simulink model "dmitry_model"  (R2022b)
settings: Solver=FixedStepDiscrete  StartTime=0.0  StopTime=10.0  FixedStep=1/ SCHED_LOOP_RATE  RelTol=1e-3
values from neighbouring files (symbols this model uses):
  g = 9.81    [startVars.m]
  KDphi = KDphi*1.0    (= 0.00082498)    [altitude_attitude_control_sim.m]
  KDpsi = KDpsi*1.0*0.8    (= 0.0004576)    [altitude_attitude_control_sim.m]
  KDtheta = KDtheta*1.4    (= 0.001977976)    [altitude_attitude_control_sim.m]
  KDz = KDz*1.0    (= 0.3498)    [altitude_attitude_control_sim.m]
  Ts = 1/SCHED_LOOP_RATE    [PitchComplementaryFilter_disc.m]    (also in RollComplementaryFilter_disc.m; YawComplementaryFilter_disc.m; altitude_attitude_control_sim.m; startVars.m)
  w_c_pitch = 0.3    [PitchComplementaryFilter_disc.m]
  w_c_roll = 0.3    [RollComplementaryFilter_disc.m]
  w_c_yaw = 55    [YawComplementaryFilter_disc.m]
  zDphi = zDphi*1.0    (= 1.31578947368)    [altitude_attitude_control_sim.m]
  zDpsi = zDpsi*1.0*1.0    (= 2.27272727273)    [altitude_attitude_control_sim.m]
  zDtheta = zDtheta*1.0    (= 1.31578947368)    [altitude_attitude_control_sim.m]
  zDz = zDz*1.0    (= 3.0303030303)    [altitude_attitude_control_sim.m]
undefined symbols (not defined in the file or in its folder): Controller, den_pitch_disc, den_roll_disc, den_yaw_disc, num_pitch_disc, num_roll_disc, num_yaw_disc, Vehicle
libraries: cstblocks x9
settings Model: ParamWorkspaceSource=ReferencedWorkspace  Creator=joseph  LastModifiedBy=Joseph
settings OptimizationCC: EnhancedBackFolding=on  PassReuseOutputArgsAs=Individual arguments  ZeroExternalMemoryAtStartup=off  ZeroInternalMemoryAtStartup=off  OptimizeBlockOrder=speed  DifferentSizesBufferReuse=on  OptimizationCustomize=off  EfficientTunableParamExpr=on
settings DebuggingCC: ParameterTunabilityLossMsg=error
settings HardwareCC: ProdBitPerPointer=32  ProdBitPerSizeT=32  ProdBitPerPtrDiffT=32  ProdLargestAtomicInteger=Long  ProdLargestAtomicFloat=Double  ProdWordSize=32  ProdHWDeviceType=ARM Compatible->ARM Cortex-M
settings SFSimCC: MATLABDynamicMemAlloc=off
settings RTWCC: Description=Embedded Coder  SystemTargetFile=ert.tlc  GenCodeOnly=on  PackageGeneratedCodeAndArtifacts=on  TemplateMakefile=ert_default_tmf  Toolchain=MinGW64 | gmake (64-bit Windows)  TargetLang=C++
settings CodeAppCC: ForceParamTrailComments=on  IgnoreCustomStorageClasses=off  OperatorAnnotations=on  SimulinkDataObjDesc=on  SFDataObjDesc=on  InsertBlockDesc=on
settings ERTTargetCC: TargetLangStandard=C++11 (ISO)  GenerateSampleERTMain=on  CodeInterfacePackaging=C++ class  RootIOFormat=Structure reference  ERTCustomFileTemplate=example_file_process.tlc

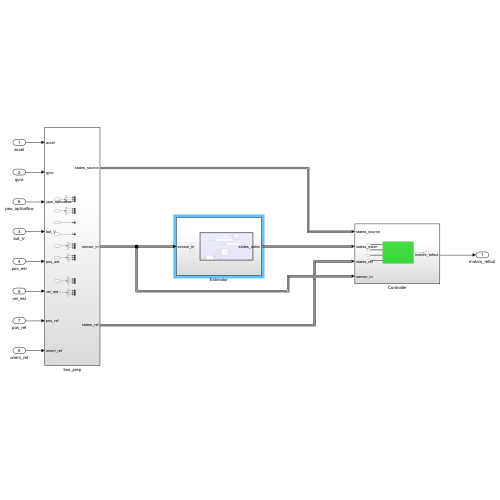
[thumbnail: Simulink's stored preview of the top-level diagram]
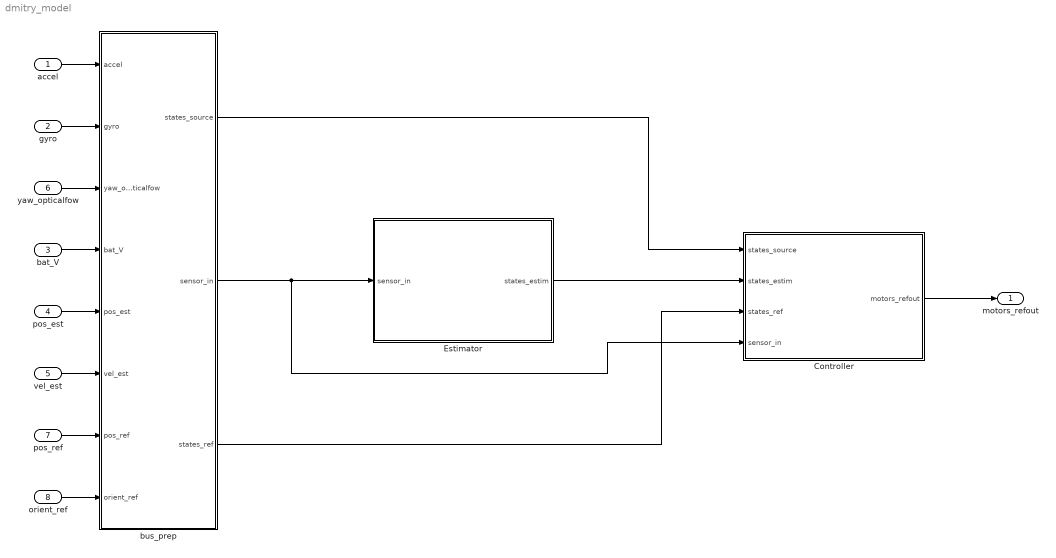
== system dmitry_model ==
  accel : Inport  OutDataTypeStr=single
  gyro : Inport  Port=2  OutDataTypeStr=single
  bat_V : Inport  Port=3  OutDataTypeStr=single
  pos_est : Inport  Port=4  OutDataTypeStr=single
  vel_est : Inport  Port=5  OutDataTypeStr=single
  yaw_opticalfow : Inport  Port=6  OutDataTypeStr=single
  pos_ref : Inport  Port=7  OutDataTypeStr=single
  orient_ref : Inport  Port=8  OutDataTypeStr=single
  Controller : Subsystem
  Estimator : Subsystem
  bus_prep : Subsystem
  motors_refout : Outport
  wires:
  accel/1 -> bus_prep/1(accel)
  gyro/1 -> bus_prep/2(gyro)
  yaw_opticalfow/1 -> bus_prep/3(yaw_opticalfow)
  bat_V/1 -> bus_prep/4(bat_V)
  pos_est/1 -> bus_prep/5(pos_est)
  vel_est/1 -> bus_prep/6(vel_est)
  pos_ref/1 -> bus_prep/7(pos_ref)
  orient_ref/1 -> bus_prep/8(orient_ref)
  bus_prep/2(sensor_in) -> Controller/4(sensor_in), Estimator/1(sensor_in)
  bus_prep/1(states_source) -> Controller/1(states_source)
  Estimator/1(states_estim) -> Controller/2(states_estim)
  Controller/1(motors_refout) -> motors_refout/1
  bus_prep/3(states_ref) -> Controller/3(states_ref)

== system dmitry_model/Controller ==
  states_source : Inport
  states_estim : Inport  Port=2
  states_ref : Inport  Port=3
  sensor_in : Inport  Port=4
  Flight Controller : Subsystem
  motors_refout : Outport
  wires:
  Flight Controller/1(motors_refout) -> motors_refout/1
  states_ref/1 -> Flight Controller/3(states_ref)
  states_estim/1 -> Flight Controller/2(states_est)
  states_source/1 -> Flight Controller/1(states_source)
  sensor_in/1 -> Flight Controller/4(sensor_in)

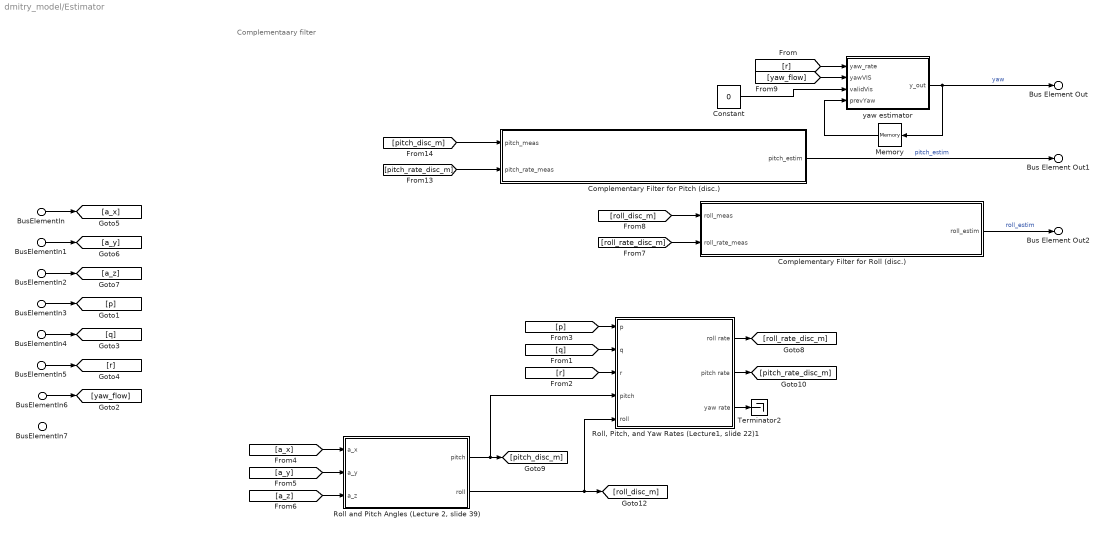
== system dmitry_model/Estimator ==
  note: Complementaary filter
  BusElementIn : Inport  PortName=sensor_in  Element=a_x
  BusElementIn1 : Inport  PortName=sensor_in  Element=a_y
  BusElementIn2 : Inport  PortName=sensor_in  Element=a_z
  BusElementIn3 : Inport  PortName=sensor_in  Element=p
  BusElementIn4 : Inport  PortName=sensor_in  Element=q
  BusElementIn5 : Inport  PortName=sensor_in  Element=r
  BusElementIn6 : Inport  PortName=sensor_in  Element=yaw_flow
  BusElementIn7 : Inport  PortName=sensor_in  Element=yaw_flow
  Complementary Filter for Pitch (disc.) : Subsystem
  Complementary Filter for Roll (disc.) : Subsystem
  Constant : Constant  Value=0
  Memory : Memory
  "Roll and Pitch Angles (Lecture 2, slide 39)" : Subsystem
  "Roll, Pitch, and Yaw Rates (Lecture1, slide 22)1" : Subsystem
  Terminator2 : Terminator
  yaw estimator : Subsystem
  Bus Element Out : Outport  PortName=states_estim  Element=yaw
  Bus Element Out1 : Outport  PortName=states_estim  Element=pitch
  Bus Element Out2 : Outport  PortName=states_estim  Element=roll
  wires:
  [a_y] -> "Roll and Pitch Angles (Lecture 2, slide 39)"/2(a_y)
  [p] -> "Roll, Pitch, and Yaw Rates (Lecture1, slide 22)1"/1(p)
  [a_x] -> "Roll and Pitch Angles (Lecture 2, slide 39)"/1(a_x)
  "Roll and Pitch Angles (Lecture 2, slide 39)"/2(roll) -> "Roll, Pitch, and Yaw Rates (Lecture1, slide 22)1"/5(roll), [roll_disc_m]
  [a_z] -> "Roll and Pitch Angles (Lecture 2, slide 39)"/3(a_z)
  "Roll and Pitch Angles (Lecture 2, slide 39)"/1(pitch) -> [pitch_disc_m], "Roll, Pitch, and Yaw Rates (Lecture1, slide 22)1"/4(pitch)
  Constant/1 -> yaw estimator/3(validVis)
  [roll_rate_disc_m] -> Complementary Filter for Roll (disc.)/2(roll_rate_meas)
  [roll_disc_m] -> Complementary Filter for Roll (disc.)/1(roll_meas)
  Complementary Filter for Roll (disc.)/1(roll_estim) -> Bus Element Out2/1  "roll_estim"
  [q] -> "Roll, Pitch, and Yaw Rates (Lecture1, slide 22)1"/2(q)
  "Roll, Pitch, and Yaw Rates (Lecture1, slide 22)1"/3(yaw rate) -> Terminator2/1
  "Roll, Pitch, and Yaw Rates (Lecture1, slide 22)1"/2(pitch rate) -> [pitch_rate_disc_m]
  Complementary Filter for Pitch (disc.)/1(pitch_estim) -> Bus Element Out1/1  "pitch_estim"
  [r] -> "Roll, Pitch, and Yaw Rates (Lecture1, slide 22)1"/3(r)
  [yaw_flow] -> yaw estimator/2(yawVIS)
  [pitch_disc_m] -> Complementary Filter for Pitch (disc.)/1(pitch_meas)
  Memory/1 -> yaw estimator/4(prevYaw)
  [pitch_rate_disc_m] -> Complementary Filter for Pitch (disc.)/2(pitch_rate_meas)
  yaw estimator/1(y_out) -> Bus Element Out/1, Memory/1  "yaw"
  "Roll, Pitch, and Yaw Rates (Lecture1, slide 22)1"/1(roll rate) -> [roll_rate_disc_m]
  [r] -> yaw estimator/1(yaw_rate)
  BusElementIn3/1 -> [p]
  BusElementIn4/1 -> [q]
  BusElementIn5/1 -> [r]
  BusElementIn/1 -> [a_x]
  BusElementIn1/1 -> [a_y]
  BusElementIn2/1 -> [a_z]
  BusElementIn6/1 -> [yaw_flow]

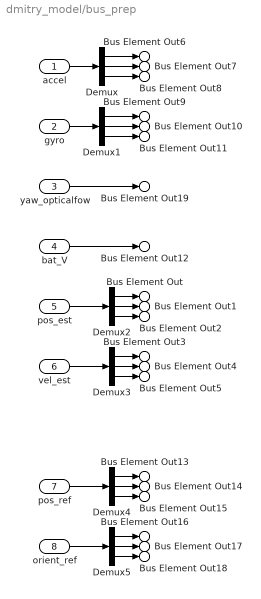
== system dmitry_model/bus_prep ==
  accel : Inport  OutDataTypeStr=single
  gyro : Inport  Port=2  OutDataTypeStr=single
  yaw_opticalfow : Inport  Port=3  OutDataTypeStr=single
  bat_V : Inport  Port=4  OutDataTypeStr=single
  pos_est : Inport  Port=5  OutDataTypeStr=single
  vel_est : Inport  Port=6  OutDataTypeStr=single
  pos_ref : Inport  Port=7  OutDataTypeStr=single
  orient_ref : Inport  Port=8  OutDataTypeStr=single
  Demux{,1..5} (6 alike) : Demux  Outputs=3
  Bus Element Out : Outport  PortName=states_source  Element=x
  Bus Element Out1 : Outport  PortName=states_source  Element=y
  Bus Element Out2 : Outport  PortName=states_source  Element=z
  Bus Element Out3 : Outport  PortName=states_source  Element=dx
  Bus Element Out4 : Outport  PortName=states_source  Element=dy
  Bus Element Out5 : Outport  PortName=states_source  Element=dz
  Bus Element Out6 : Outport  Port=2  PortName=sensor_in  Element=a_x
  Bus Element Out7 : Outport  Port=2  PortName=sensor_in  Element=a_y
  Bus Element Out8 : Outport  Port=2  PortName=sensor_in  Element=a_z
  Bus Element Out9 : Outport  Port=2  PortName=sensor_in  Element=p
  Bus Element Out10 : Outport  Port=2  PortName=sensor_in  Element=q
  Bus Element Out11 : Outport  Port=2  PortName=sensor_in  Element=r
  Bus Element Out12 : Outport  Port=2  PortName=sensor_in  Element=V_batt
  Bus Element Out19 : Outport  Port=2  PortName=sensor_in  Element=yaw_flow
  Bus Element Out13 : Outport  Port=3  PortName=states_ref  Element=x
  Bus Element Out14 : Outport  Port=3  PortName=states_ref  Element=y
  Bus Element Out15 : Outport  Port=3  PortName=states_ref  Element=z
  Bus Element Out16 : Outport  Port=3  PortName=states_ref  Element=yaw
  Bus Element Out17 : Outport  Port=3  PortName=states_ref  Element=pitch
  Bus Element Out18 : Outport  Port=3  PortName=states_ref  Element=roll
  wires:
  pos_ref/1 -> Demux4/1
  orient_ref/1 -> Demux5/1
  pos_est/1 -> Demux2/1
  Demux3/1 -> Bus Element Out3/1
  Demux3/3 -> Bus Element Out5/1
  Demux5/3 -> Bus Element Out18/1
  vel_est/1 -> Demux3/1
  accel/1 -> Demux/1
  gyro/1 -> Demux1/1
  Demux5/1 -> Bus Element Out16/1
  Demux4/1 -> Bus Element Out13/1
  Demux1/1 -> Bus Element Out9/1
  Demux3/2 -> Bus Element Out4/1
  Demux4/2 -> Bus Element Out14/1
  Demux2/2 -> Bus Element Out1/1
  Demux1/3 -> Bus Element Out11/1
  Demux5/2 -> Bus Element Out17/1
  Demux4/3 -> Bus Element Out15/1
  Demux2/1 -> Bus Element Out/1
  Demux/3 -> Bus Element Out8/1
  Demux/1 -> Bus Element Out6/1
  Demux2/3 -> Bus Element Out2/1
  Demux1/2 -> Bus Element Out10/1
  yaw_opticalfow/1 -> Bus Element Out19/1
  bat_V/1 -> Bus Element Out12/1
  Demux/2 -> Bus Element Out7/1

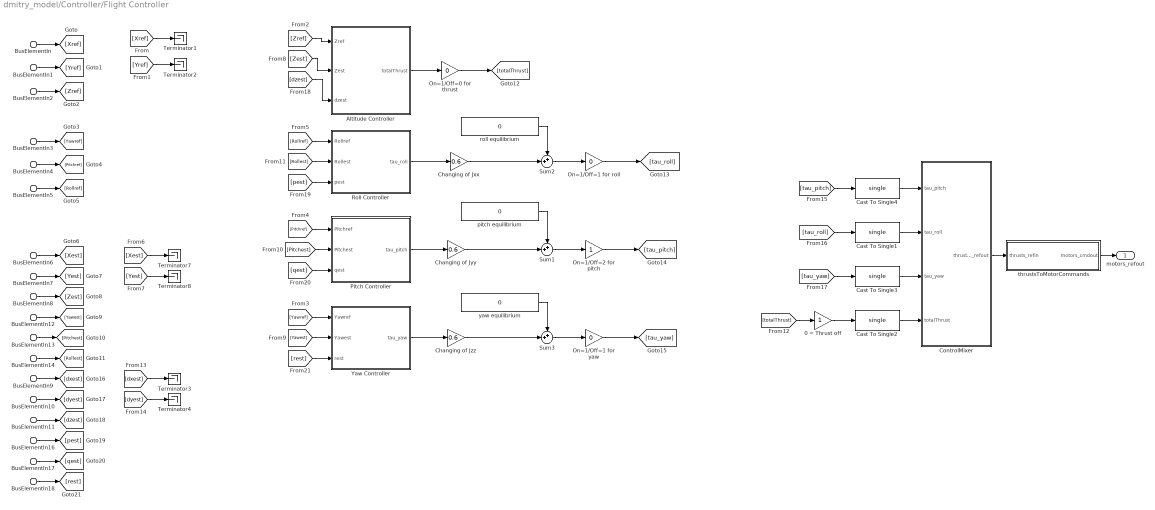
== system dmitry_model/Controller/Flight Controller ==
  BusElementIn6 : Inport  PortName=states_source  Element=x
  BusElementIn7 : Inport  PortName=states_source  Element=y
  BusElementIn8 : Inport  PortName=states_source  Element=z
  BusElementIn9 : Inport  PortName=states_source  Element=dx
  BusElementIn10 : Inport  PortName=states_source  Element=dy
  BusElementIn11 : Inport  PortName=states_source  Element=dz
  BusElementIn12 : Inport  Port=2  PortName=states_est  Element=yaw
  BusElementIn13 : Inport  Port=2  PortName=states_est  Element=pitch
  BusElementIn14 : Inport  Port=2  PortName=states_est  Element=roll
  BusElementIn : Inport  Port=3  PortName=states_ref  Element=x
  BusElementIn1 : Inport  Port=3  PortName=states_ref  Element=y
  BusElementIn2 : Inport  Port=3  PortName=states_ref  Element=z
  BusElementIn3 : Inport  Port=3  PortName=states_ref  Element=yaw
  BusElementIn4 : Inport  Port=3  PortName=states_ref  Element=pitch
  BusElementIn5 : Inport  Port=3  PortName=states_ref  Element=roll
  BusElementIn16 : Inport  Port=4  PortName=sensor_in  Element=p
  BusElementIn17 : Inport  Port=4  PortName=sensor_in  Element=q
  BusElementIn18 : Inport  Port=4  PortName=sensor_in  Element=r
  0 = Thrust off : Gain
  Altitude Controller : Subsystem
  Cast To Single{1..4} (4 alike) : DataTypeConversion  OutDataTypeStr=single  SaturateOnIntegerOverflow=off  RndMeth=Floor
  Changing of Jxx : Gain  Gain=0.6
  Changing of Jyy : Gain  Gain=0.6
  Changing of Jzz : Gain  Gain=0.6
  ControlMixer : Subsystem
  On=1/Off=0 for thrust : Gain  Gain=0
  On=1/Off=1 for roll : Gain  Gain=0
  On=1/Off=1 for yaw : Gain  Gain=0
  On=1/Off=2 for pitch : Gain
  Pitch Controller : Subsystem
  Roll Controller : Subsystem
  Sum1 : Sum  Inputs=++|
  Sum2 : Sum  Inputs=++|
  Sum3 : Sum  Inputs=++|
  Terminator{1..4,7..8} (6 alike) : Terminator
  Yaw Controller : Subsystem
  pitch equilibrium : Constant  Value=0  SampleTime=Ts
  roll equilibrium : Constant  Value=0  SampleTime=Ts
  thrustsToMotorCommands : Subsystem
  yaw equilibrium : Constant  Value=0  SampleTime=Ts
  motors_refout : Outport  VectorParamsAs1DForOutWhenUnconnected=off
  wires:
  ControlMixer/1(thrusts_refout) -> thrustsToMotorCommands/1(thrusts_refin)
  thrustsToMotorCommands/1(motors_cmdout) -> motors_refout/1
  Cast To Single1/1 -> ControlMixer/2(tau_roll)
  [tau_roll] -> Cast To Single1/1
  Cast To Single2/1 -> ControlMixer/4(totalThrust)
  BusElementIn/1 -> [Xref]
  BusElementIn1/1 -> [Yref]
  BusElementIn2/1 -> [Zref]
  BusElementIn5/1 -> [Rollref]
  BusElementIn4/1 -> [Pitchref]
  BusElementIn3/1 -> [Yawref]
  [Xref] -> Terminator1/1
  [Yref] -> Terminator2/1
  [Zref] -> Altitude Controller/1(Zref)
  BusElementIn6/1 -> [Xest]
  BusElementIn7/1 -> [Yest]
  BusElementIn8/1 -> [Zest]
  BusElementIn12/1 -> [Yawest]
  BusElementIn13/1 -> [Pitchest]
  BusElementIn14/1 -> [Rollest]
  [Zest] -> Altitude Controller/2(Zest)
  [Yest] -> Terminator8/1
  [Xest] -> Terminator7/1
  Altitude Controller/1(totalThrust) -> On=1/Off=0 for thrust/1
  On=1/Off=0 for thrust/1 -> [totalThrust]
  [totalThrust] -> 0 = Thrust off/1
  Roll Controller/1(tau_roll) -> Changing of Jxx/1
  [tau_yaw] -> Cast To Single3/1
  Cast To Single3/1 -> ControlMixer/3(tau_yaw)
  [tau_pitch] -> Cast To Single4/1
  Cast To Single4/1 -> ControlMixer/1(tau_pitch)
  [Rollref] -> Roll Controller/1(Rollref)
  [Rollest] -> Roll Controller/2(Rollest)
  Pitch Controller/1(tau_pitch) -> Changing of Jyy/1
  [Pitchest] -> Pitch Controller/2(Pitchest)
  [Pitchref] -> Pitch Controller/1(Pitchref)
  Yaw Controller/1(tau_yaw) -> Changing of Jzz/1
  [Yawref] -> Yaw Controller/1(Yawref)
  [Yawest] -> Yaw Controller/2(Yawest)
  BusElementIn9/1 -> [dxest]
  BusElementIn10/1 -> [dyest]
  BusElementIn11/1 -> [dzest]
  BusElementIn16/1 -> [pest]
  BusElementIn17/1 -> [qest]
  BusElementIn18/1 -> [rest]
  [dxest] -> Terminator3/1
  [dyest] -> Terminator4/1
  [pest] -> Roll Controller/3(pest)
  [dzest] -> Altitude Controller/3(dzest)
  [qest] -> Pitch Controller/3(qest)
  [rest] -> Yaw Controller/3(rest)
  roll equilibrium/1 -> Sum2/1
  Changing of Jxx/1 -> Sum2/2
  pitch equilibrium/1 -> Sum1/1
  yaw equilibrium/1 -> Sum3/1
  Changing of Jyy/1 -> Sum1/2
  Changing of Jzz/1 -> Sum3/2
  Sum3/1 -> On=1/Off=1 for yaw/1
  Sum1/1 -> On=1/Off=2 for pitch/1
  Sum2/1 -> On=1/Off=1 for roll/1
  On=1/Off=1 for roll/1 -> [tau_roll]
  On=1/Off=2 for pitch/1 -> [tau_pitch]
  On=1/Off=1 for yaw/1 -> [tau_yaw]
  0 = Thrust off/1 -> Cast To Single2/1

== system dmitry_model/Estimator/Complementary Filter for Pitch (disc.) ==
  pitch_meas : Inport
  pitch_rate_meas : Inport  Port=2
  Discrete Transfer Fcn : DiscreteTransferFcn  Numerator=[num_pitch_disc]  Denominator=[den_pitch_disc]  SampleTime=Ts
  Gain : Gain  Gain=w_c_pitch
  Sum : Sum  Inputs=+|+
  pitch_estim : Outport
  wires:
  Sum/1 -> Discrete Transfer Fcn/1
  Gain/1 -> Sum/1
  pitch_rate_meas/1 -> Sum/2
  pitch_meas/1 -> Gain/1
  Discrete Transfer Fcn/1 -> pitch_estim/1  "pitch_estim"

== system dmitry_model/Estimator/Complementary Filter for Roll (disc.) ==
  roll_meas : Inport
  roll_rate_meas : Inport  Port=2
  Discrete Transfer Fcn : DiscreteTransferFcn  Numerator=[num_roll_disc]  Denominator=[den_roll_disc]  SampleTime=Ts
  Gain : Gain  Gain=w_c_roll
  Sum : Sum  Inputs=+|+
  roll_estim : Outport
  wires:
  Discrete Transfer Fcn/1 -> roll_estim/1  "roll_estim"
  roll_meas/1 -> Gain/1
  roll_rate_meas/1 -> Sum/2
  Gain/1 -> Sum/1
  Sum/1 -> Discrete Transfer Fcn/1

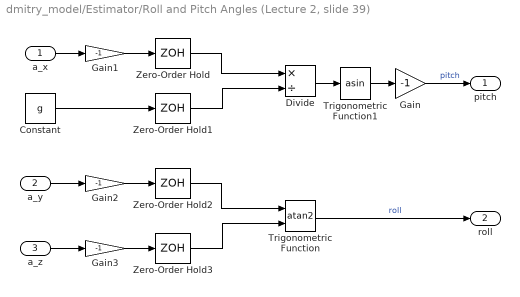
== system dmitry_model/Estimator/Roll and Pitch Angles (Lecture 2, slide 39) ==
  a_x : Inport
  a_y : Inport  Port=2
  a_z : Inport  Port=3
  Constant : Constant  Value=g
  Divide : Product  Inputs=*/
  Gain{,1..3} (4 alike) : Gain  Gain=-1
  Trigonometric Function : Trigonometry  Operator=atan2
  Trigonometric Function1 : Trigonometry  Operator=asin
  Zero-Order Hold{,1..3} (4 alike) : ZeroOrderHold  SampleTime=Ts
  pitch : Outport
  roll : Outport  Port=2
  wires:
  Gain/1 -> pitch/1  "pitch"
  Trigonometric Function/1 -> roll/1  "roll"
  a_y/1 -> Gain2/1
  a_z/1 -> Gain3/1
  a_x/1 -> Gain1/1
  Constant/1 -> Zero-Order Hold1/1
  Trigonometric Function1/1 -> Gain/1
  Divide/1 -> Trigonometric Function1/1
  Zero-Order Hold/1 -> Divide/1
  Zero-Order Hold1/1 -> Divide/2
  Zero-Order Hold2/1 -> Trigonometric Function/1
  Zero-Order Hold3/1 -> Trigonometric Function/2
  Gain1/1 -> Zero-Order Hold/1
  Gain2/1 -> Zero-Order Hold2/1
  Gain3/1 -> Zero-Order Hold3/1

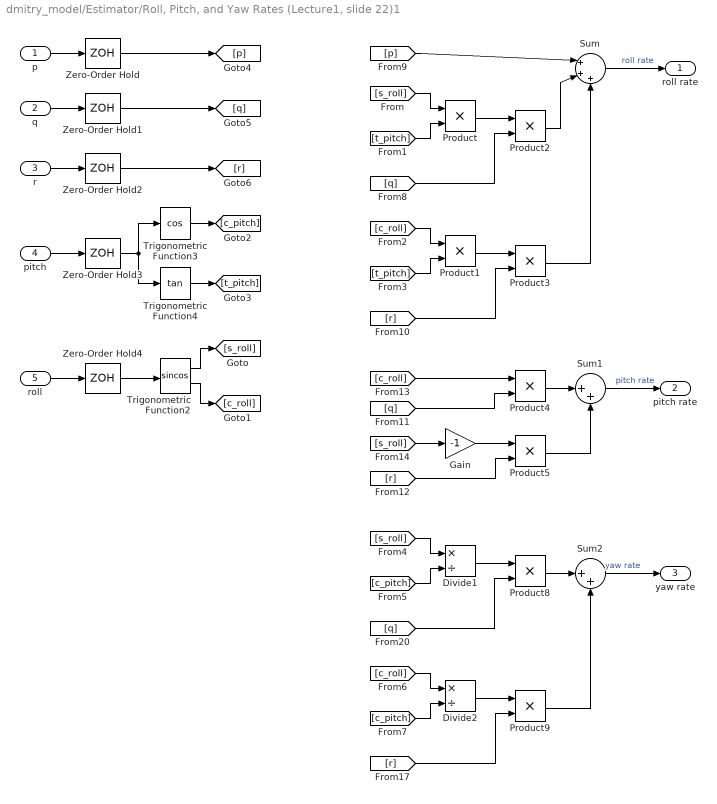
== system dmitry_model/Estimator/Roll, Pitch, and Yaw Rates (Lecture1, slide 22)1 ==
  p : Inport
  q : Inport  Port=2
  r : Inport  Port=3
  pitch : Inport  Port=4
  roll : Inport  Port=5
  Divide1 : Product  Inputs=*/
  Divide2 : Product  Inputs=*/
  Gain : Gain  Gain=-1
  Product{,1..5,8..9} (8 alike) : Product
  Sum : Sum  Inputs=|+++
  Sum1 : Sum  Inputs=|++
  Sum2 : Sum  Inputs=|++
  Trigonometric Function2 : Trigonometry  Operator=sincos
  Trigonometric Function3 : Trigonometry  Operator=cos
  Trigonometric Function4 : Trigonometry  Operator=tan
  Zero-Order Hold{,1..4} (5 alike) : ZeroOrderHold  SampleTime=Ts
  roll rate : Outport
  pitch rate : Outport  Port=2
  yaw rate : Outport  Port=3
  wires:
  roll/1 -> Zero-Order Hold4/1
  Trigonometric Function2/1 -> [s_roll]
  Trigonometric Function2/2 -> [c_roll]
  pitch/1 -> Zero-Order Hold3/1
  Trigonometric Function4/1 -> [t_pitch]
  Trigonometric Function3/1 -> [c_pitch]
  [s_roll] -> Product/1
  [t_pitch] -> Product/2
  [t_pitch] -> Product1/2
  [c_roll] -> Product1/1
  [s_roll] -> Divide1/1
  [c_pitch] -> Divide1/2
  [c_pitch] -> Divide2/2
  [c_roll] -> Divide2/1
  p/1 -> Zero-Order Hold/1
  q/1 -> Zero-Order Hold1/1
  r/1 -> Zero-Order Hold2/1
  [q] -> Product2/2
  Product/1 -> Product2/1
  Sum/1 -> roll rate/1  "roll rate"
  [p] -> Sum/1
  Product1/1 -> Product3/1
  [r] -> Product3/2
  Product2/1 -> Sum/2
  Product3/1 -> Sum/3
  [r] -> Product5/2
  Gain/1 -> Product5/1
  Sum1/1 -> pitch rate/1  "pitch rate"
  [c_roll] -> Product4/1
  [q] -> Product4/2
  [s_roll] -> Gain/1
  Product4/1 -> Sum1/1
  Product5/1 -> Sum1/2
  [r] -> Product9/2
  Divide2/1 -> Product9/1
  Divide1/1 -> Product8/1
  [q] -> Product8/2
  Sum2/1 -> yaw rate/1  "yaw rate"
  Product8/1 -> Sum2/1
  Product9/1 -> Sum2/2
  Zero-Order Hold/1 -> [p]
  Zero-Order Hold1/1 -> [q]
  Zero-Order Hold2/1 -> [r]
  Zero-Order Hold3/1 -> Trigonometric Function4/1, Trigonometric Function3/1
  Zero-Order Hold4/1 -> Trigonometric Function2/1

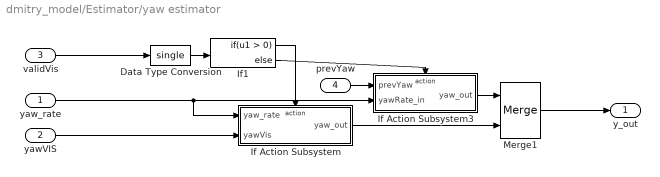
== system dmitry_model/Estimator/yaw estimator ==
  yaw_rate : Inport
  yawVIS : Inport  Port=2
  validVis : Inport  Port=3
  prevYaw : Inport  Port=4
  Data Type Conversion : DataTypeConversion  OutDataTypeStr=single  SaturateOnIntegerOverflow=off  RndMeth=Floor
  If Action Subsystem3 : Subsystem  TreatAsAtomicUnit=on
  If Action Subsystem : Subsystem  TreatAsAtomicUnit=on
  If1 : If
  Merge1 : Merge
  y_out : Outport
  wires:
  If Action Subsystem/1(yaw_out) -> Merge1/2
  Merge1/1 -> y_out/1
  yawVIS/1 -> If Action Subsystem/2(yawVis)
  Data Type Conversion/1 -> If1/1
  validVis/1 -> Data Type Conversion/1
  yaw_rate/1 -> If Action Subsystem/1(yaw_rate), If Action Subsystem3/2(yawRate_in)
  If Action Subsystem3/1(yaw_out) -> Merge1/1
  If1/2 -> If Action Subsystem3/Action
  If1/1 -> If Action Subsystem/Action
  prevYaw/1 -> If Action Subsystem3/1(prevYaw)

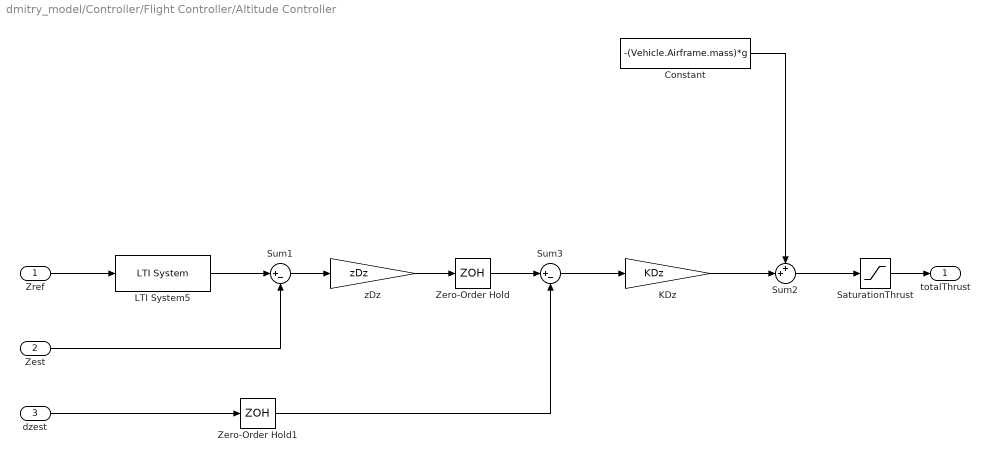
== system dmitry_model/Controller/Flight Controller/Altitude Controller ==
  Zref : Inport
  Zest : Inport  Port=2
  dzest : Inport  Port=3
  Constant : Constant  Value=-(Vehicle.Airframe.mass)*g  SampleTime=Ts
  KDz : Gain  Gain=KDz
  LTI System5 : cstblocks/LTI System  sys=F_discr  IC=[]
  SaturationThrust : Saturate  UpperLimit=4*Controller.totalThrustMaxRelative*Controller.motorsThrustPerMotorMax  LowerLimit=-4*Controller.totalThrustMaxRelative*Controller.motorsThrustPerMotorMax  OutDataTypeStr=single
  Sum1 : Sum  Inputs=|+-
  Sum2 : Sum  Inputs=++|
  Sum3 : Sum  Inputs=|+-
  Zero-Order Hold : ZeroOrderHold  SampleTime=Ts
  Zero-Order Hold1 : ZeroOrderHold  SampleTime=Ts
  zDz : Gain  Gain=zDz
  totalThrust : Outport
  wires:
  Zest/1 -> Sum1/2
  Constant/1 -> Sum2/1
  SaturationThrust/1 -> totalThrust/1
  Sum1/1 -> zDz/1
  zDz/1 -> Zero-Order Hold/1
  Sum3/1 -> KDz/1
  dzest/1 -> Zero-Order Hold1/1
  Zero-Order Hold1/1 -> Sum3/2
  Sum2/1 -> SaturationThrust/1
  Zref/1 -> LTI System5/1
  LTI System5/1 -> Sum1/1
  Zero-Order Hold/1 -> Sum3/1
  KDz/1 -> Sum2/2

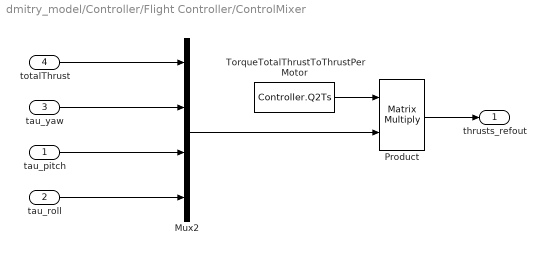
== system dmitry_model/Controller/Flight Controller/ControlMixer ==
  tau_pitch : Inport
  tau_roll : Inport  Port=2
  tau_yaw : Inport  Port=3
  totalThrust : Inport  Port=4
  Mux2 : Mux
  Product : Product  Multiplication=Matrix(*)  RndMeth=Zero
  TorqueTotalThrustToThrustPerMotor : Constant  Value=Controller.Q2Ts  OutDataTypeStr=single
  thrusts_refout : Outport  VectorParamsAs1DForOutWhenUnconnected=off
  wires:
  Product/1 -> thrusts_refout/1
  tau_roll/1 -> Mux2/4
  tau_pitch/1 -> Mux2/3
  tau_yaw/1 -> Mux2/2
  totalThrust/1 -> Mux2/1
  TorqueTotalThrustToThrustPerMotor/1 -> Product/1
  Mux2/1 -> Product/2

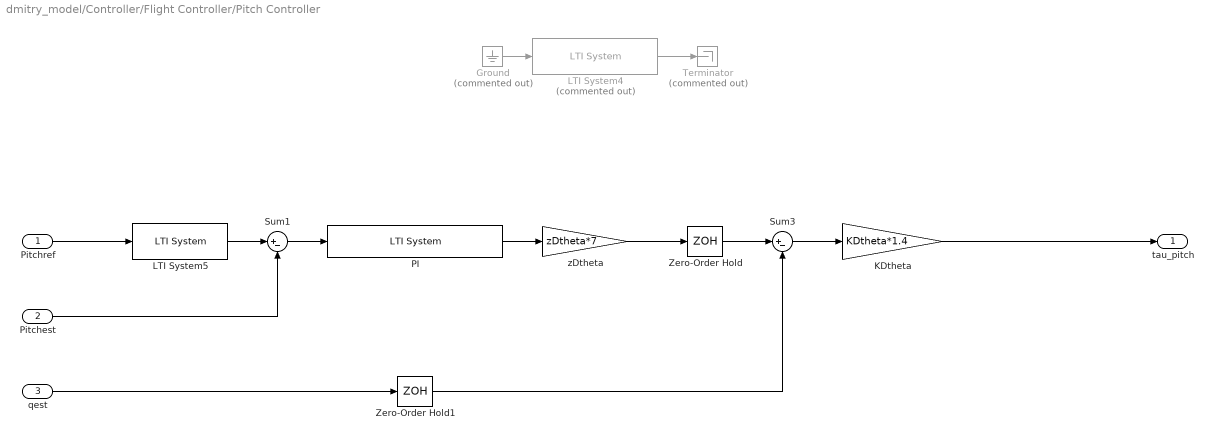
== system dmitry_model/Controller/Flight Controller/Pitch Controller ==
  Pitchref : Inport
  Pitchest : Inport  Port=2
  qest : Inport  Port=3
  Ground : Ground  Commented=on
  KDtheta : Gain  Gain=KDtheta*1.4
  LTI System4 : cstblocks/LTI System  Commented=on  sys=Ctheta_causal_discr  IC=[]
  LTI System5 : cstblocks/LTI System  sys=F_discr  IC=[]
  PI : cstblocks/LTI System  sys=Ctheta_2DOF_inegral_causal_discr  IC=[]
  Sum1 : Sum  Inputs=|+-
  Sum3 : Sum  Inputs=|+-
  Terminator : Terminator  Commented=on
  Zero-Order Hold : ZeroOrderHold  SampleTime=Ts
  Zero-Order Hold1 : ZeroOrderHold  SampleTime=Ts
  zDtheta : Gain  Gain=zDtheta*7
  tau_pitch : Outport
  wires:
  LTI System5/1 -> Sum1/1
  Pitchest/1 -> Sum1/2
  Pitchref/1 -> LTI System5/1
  KDtheta/1 -> tau_pitch/1
  Ground/1 -> LTI System4/1
  LTI System4/1 -> Terminator/1
  Sum1/1 -> PI/1
  zDtheta/1 -> Zero-Order Hold/1
  PI/1 -> zDtheta/1
  qest/1 -> Zero-Order Hold1/1
  Zero-Order Hold1/1 -> Sum3/2
  Sum3/1 -> KDtheta/1
  Zero-Order Hold/1 -> Sum3/1

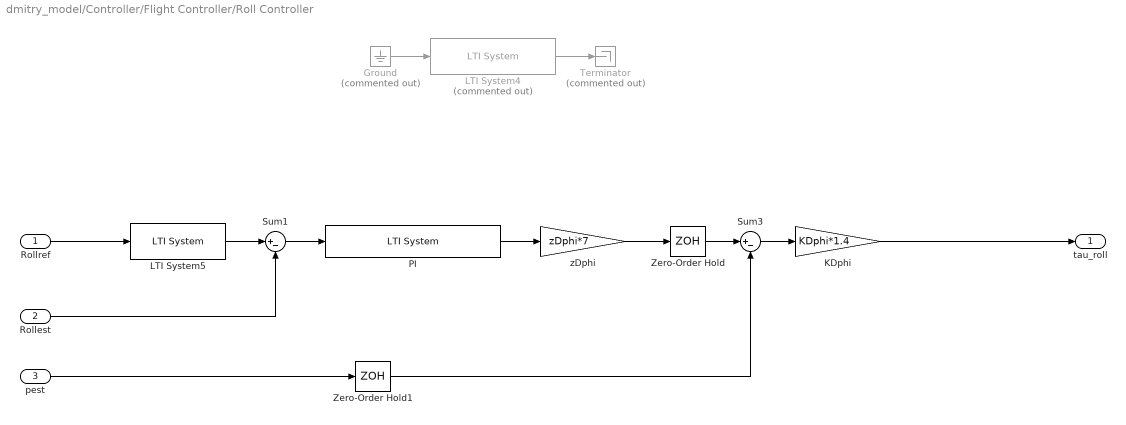
== system dmitry_model/Controller/Flight Controller/Roll Controller ==
  Rollref : Inport
  Rollest : Inport  Port=2
  pest : Inport  Port=3
  Ground : Ground  Commented=on
  KDphi : Gain  Gain=KDphi*1.4
  LTI System4 : cstblocks/LTI System  Commented=on  sys=Cphi_causal_discr  IC=[]
  LTI System5 : cstblocks/LTI System  sys=F_discr  IC=[]
  PI : cstblocks/LTI System  sys=Cphi_2DOF_inegral_causal_discr  IC=[]
  Sum1 : Sum  Inputs=|+-
  Sum3 : Sum  Inputs=|+-
  Terminator : Terminator  Commented=on
  Zero-Order Hold : ZeroOrderHold  SampleTime=Ts
  Zero-Order Hold1 : ZeroOrderHold  SampleTime=Ts
  zDphi : Gain  Gain=zDphi*7
  tau_roll : Outport
  wires:
  KDphi/1 -> tau_roll/1
  Rollref/1 -> LTI System5/1
  Rollest/1 -> Sum1/2
  LTI System5/1 -> Sum1/1
  Ground/1 -> LTI System4/1
  LTI System4/1 -> Terminator/1
  Sum1/1 -> PI/1
  PI/1 -> zDphi/1
  zDphi/1 -> Zero-Order Hold/1
  pest/1 -> Zero-Order Hold1/1
  Sum3/1 -> KDphi/1
  Zero-Order Hold1/1 -> Sum3/2
  Zero-Order Hold/1 -> Sum3/1

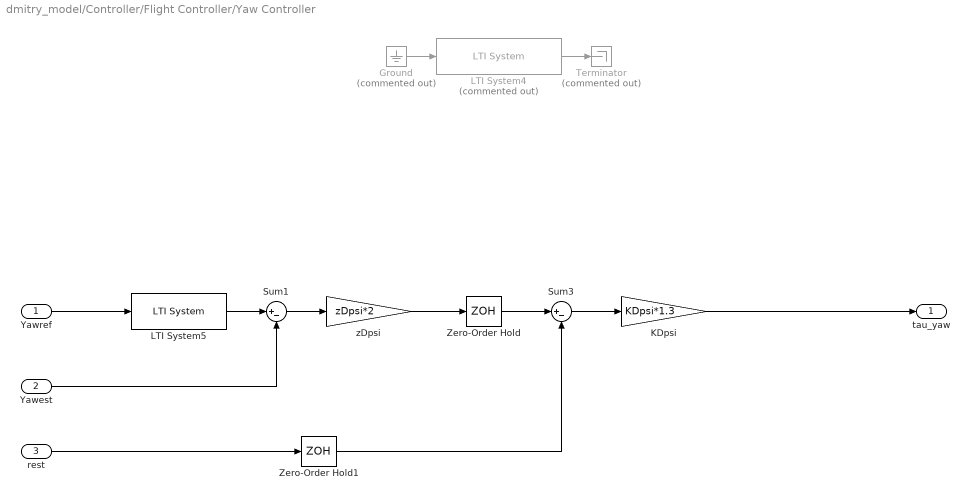
== system dmitry_model/Controller/Flight Controller/Yaw Controller ==
  Yawref : Inport
  Yawest : Inport  Port=2
  rest : Inport  Port=3
  Ground : Ground  Commented=on
  KDpsi : Gain  Gain=KDpsi*1.3
  LTI System4 : cstblocks/LTI System  Commented=on  sys=Cpsi_causal_discr  IC=[]
  LTI System5 : cstblocks/LTI System  sys=F_discr  IC=[]
  Sum1 : Sum  Inputs=|+-
  Sum3 : Sum  Inputs=|+-
  Terminator : Terminator  Commented=on
  Zero-Order Hold : ZeroOrderHold  SampleTime=Ts
  Zero-Order Hold1 : ZeroOrderHold  SampleTime=Ts
  zDpsi : Gain  Gain=zDpsi*2
  tau_yaw : Outport
  wires:
  LTI System5/1 -> Sum1/1
  Yawest/1 -> Sum1/2
  Yawref/1 -> LTI System5/1
  KDpsi/1 -> tau_yaw/1
  Ground/1 -> LTI System4/1
  LTI System4/1 -> Terminator/1
  Sum1/1 -> zDpsi/1
  zDpsi/1 -> Zero-Order Hold/1
  rest/1 -> Zero-Order Hold1/1
  Zero-Order Hold1/1 -> Sum3/2
  Sum3/1 -> KDpsi/1
  Zero-Order Hold/1 -> Sum3/1

== system dmitry_model/Controller/Flight Controller/thrustsToMotorCommands ==
  thrusts_refin : Inport
  MotorDirections : Gain  Gain=[1 -1 1 -1]
  Saturation5 : Saturate  UpperLimit=Vehicle.Motor.maxLimit  LowerLimit=Vehicle.Motor.minLimit
  ThrustToMotorCommand : Gain  Gain=-Vehicle.Motor.thrustToMotorCommand
  motors_cmdout : Outport  VectorParamsAs1DForOutWhenUnconnected=off
  wires:
  Saturation5/1 -> MotorDirections/1
  MotorDirections/1 -> motors_cmdout/1
  ThrustToMotorCommand/1 -> Saturation5/1
  thrusts_refin/1 -> ThrustToMotorCommand/1

== system dmitry_model/Estimator/yaw estimator/If Action Subsystem3 ==
  prevYaw : Inport
  yawRate_in : Inport  Port=2
  Action Port : ActionPort  ActionPortLabel=else
  Gain : Gain  Gain=Ts
  Sum : Sum  Inputs=++|
  yaw_out : Outport  VectorParamsAs1DForOutWhenUnconnected=off
  wires:
  yawRate_in/1 -> Gain/1
  Sum/1 -> yaw_out/1
  prevYaw/1 -> Sum/1
  Gain/1 -> Sum/2

== system dmitry_model/Estimator/yaw estimator/If Action Subsystem ==
  yaw_rate : Inport
  yawVis : Inport  Port=2
  Action Port : ActionPort  ActionPortLabel=if(u1 > 0)
  Complementary Filter for Yaw (disc.) : Subsystem
  yaw_out : Outport  VectorParamsAs1DForOutWhenUnconnected=off
  wires:
  yaw_rate/1 -> Complementary Filter for Yaw (disc.)/2(yaw_rate_meas)
  yawVis/1 -> Complementary Filter for Yaw (disc.)/1(yaw_meas)
  Complementary Filter for Yaw (disc.)/1(yaw_estim) -> yaw_out/1  "yaw_estim"

== system dmitry_model/Estimator/yaw estimator/If Action Subsystem/Complementary Filter for Yaw (disc.) ==
  yaw_meas : Inport
  yaw_rate_meas : Inport  Port=2
  Discrete Transfer Fcn : DiscreteTransferFcn  Numerator=[num_yaw_disc]  Denominator=[den_yaw_disc]  SampleTime=Ts
  Gain : Gain  Gain=w_c_yaw
  Sum : Sum  Inputs=+|+
  yaw_estim : Outport
  wires:
  Discrete Transfer Fcn/1 -> yaw_estim/1  "yaw_estim"
  yaw_meas/1 -> Gain/1
  yaw_rate_meas/1 -> Sum/2
  Gain/1 -> Sum/1
  Sum/1 -> Discrete Transfer Fcn/1
